simulink model "NPNwithDDD"  (R2018a)
settings: Solver=FixedStepDiscrete  StartTime=0.0  StopTime=10000  FixedStep=1  RelTol=1e-3  EnableMultiTasking=on
libraries: model_library x4
settings Model: SnapshotInterval=1  Creator=houssamabbas  LastModifiedBy=Arsalan
settings SolverCC: AutoInsertRateTranBlk=on
settings OptimizationCC: LifeSpan=inf
settings DebuggingCC: SFUnexpectedBacktrackingDiag=warning  SFNoUnconditionalDefaultTransitionDiag=warning  SFExecutionAtInitializationDiag=none
settings CodeAppCC: StateflowObjectComments=on
settings GRTTargetCC: TargetLangStandard=C89/C90 (ANSI)
settings ConfigComp: CovMetricSettings=dw  CovHtmlReporting=on  CovSaveCumulativeToWorkspaceVar=on  CovSaveSingleToWorkspaceVar=on  CovExternalEMLEnable=off

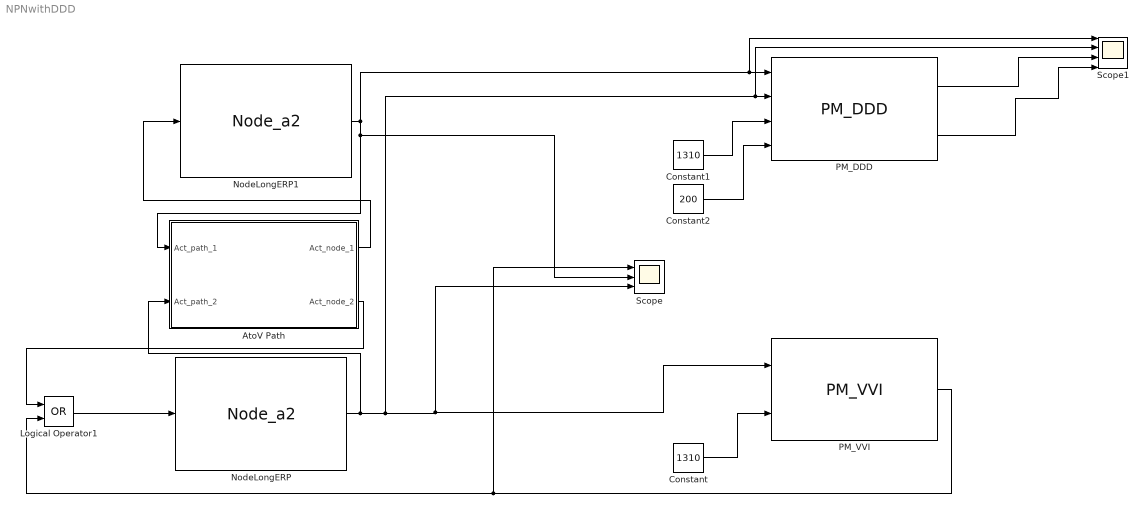
== system NPNwithDDD ==
  AtoV Path : Subsystem  AncestorBlock=model_library/Path_a2
  Constant : Constant  Value=1310  OutDataTypeStr=uint16
  Constant1 : Constant  Value=1310  OutDataTypeStr=uint16
  Constant2 : Constant  Value=200  OutDataTypeStr=uint16
  Logical Operator1 : Logic  Operator=OR  AllPortsSameDT=off  OutDataTypeStr=boolean
  NodeLongERP : model_library/Node_a2
      link override ERP_def: Value=300
      link override Rest_def: Value=2000
  NodeLongERP1 : model_library/Node_a2
      link override ERP_def: Value=300
      link override Rest_def: Value=1000
  PM_DDD : model_library/PM_DDD
  PM_VVI : model_library/PM_VVI
  Scope : Scope  NumInputPorts=3
  Scope1 : Scope  NumInputPorts=4
  wires:
  NodeLongERP1/1 -> Scope/2, AtoV Path/1(Act_path_1), Scope1/1, PM_DDD/1
  AtoV Path/2(Act_node_2) -> Logical Operator1/1
  NodeLongERP/1 -> Scope1/2, PM_DDD/2, PM_VVI/1, Scope/3, AtoV Path/2(Act_path_2)
  AtoV Path/1(Act_node_1) -> NodeLongERP1/1
  Logical Operator1/1 -> NodeLongERP/1
  PM_VVI/1 -> Scope/1, Logical Operator1/2
  Constant/1 -> PM_VVI/2
  Constant1/1 -> PM_DDD/3
  Constant2/1 -> PM_DDD/4
  PM_DDD/1 -> Scope1/3
  PM_DDD/2 -> Scope1/4

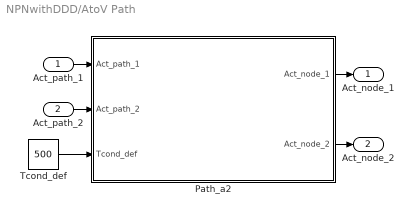
== system NPNwithDDD/AtoV Path ==
  Act_path_1 : Inport
  Act_path_2 : Inport  Port=2
  Path_a2 : Stateflow chart  TreatAsAtomicUnit=on
  Tcond_def : Constant  Value=500  OutDataTypeStr=uint16
  Act_node_1 : Outport
  Act_node_2 : Outport  Port=2
  wires:
  Tcond_def/1 -> Path_a2/3(Tcond_def)
  Path_a2/2(Act_node_2) -> Act_node_2/1
  Act_path_1/1 -> Path_a2/1(Act_path_1)
  Act_path_2/1 -> Path_a2/2(Act_path_2)
  Path_a2/1(Act_node_1) -> Act_node_1/1

== stateflow chart NPNwithDDD/AtoV Path/Path_a2 ==
  state path
    state Idle
    state Ante
    state Retro
    state Conflict
    state Double
    (default) -> Idle
    Idle -> Ante [order 1] : [Act_path_1==true]/{Tcond_cur=Tcond_def;}
    Idle -> Retro [order 2] : [Act_path_2==true]/{Tcond_cur=Tcond_def;}
    Conflict -> Idle [order 1] : [uptime>0]/{Act_node_1=false;Act_node_2=false;}
    Ante -> Ante [order 3] : [Act_path_2==false && Tcond_cur>uint16(0)]/{Tcond_cur = Tcond_cur - uint16(1);}
    Retro -> Retro [order 3] : [Act_path_1==false && Tcond_cur>uint16(0)]/{Tcond_cur = Tcond_cur - uint16(1);}
    Ante -> Double [order 2] : [Act_path_2==true]
    Ante -> Conflict [order 1] : [Act_path_2==false && Tcond_cur<=uint16(0)]/{Act_node_2=true;uptime=uint16(0);}
    Retro -> Conflict [order 1] : [Act_path_1==false && Tcond_cur<=uint16(0)]/{Act_node_1=true;uptime=uint16(0);}
    Retro -> Double [order 2] : [Act_path_1==true]
    Conflict -> Conflict [order 2] : [uptime<=uint16(0)]/{uptime = uptime + uint16(1);}
    Double -> Conflict : [Tcond_cur<=uint16(0)]/{uptime=uint16(0);}
  data: Act_path_1 input boolean; Act_path_2 input boolean; Act_node_1 output boolean; Act_node_2 output boolean; Tcond_cur local uint16; Tcond_def input uint16; uptime local uint16
